simulink model "AEB_CodeGeneration"  (R2025a)
settings: Solver=VariableStepAuto  StartTime=0.0  StopTime=10.0  RelTol=1e-3
settings Model: Creator=Rudransh  LastModifiedBy=Rudransh

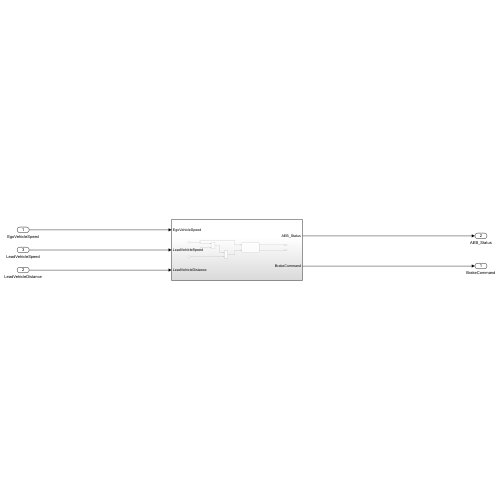
[thumbnail: Simulink's stored preview of the top-level diagram]
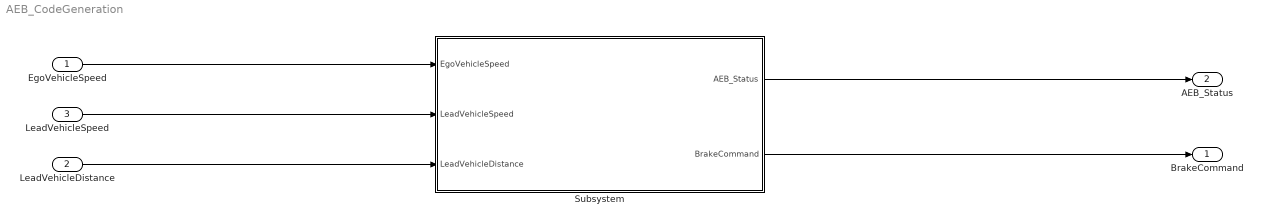
== system AEB_CodeGeneration ==
  EgoVehicleSpeed : Inport
  LeadVehicleDistance : Inport  Port=2
  LeadVehicleSpeed : Inport  Port=3
  Subsystem : Subsystem
  BrakeCommand : Outport
  AEB_Status : Outport  Port=2
  wires:
  EgoVehicleSpeed/1 -> Subsystem/1(EgoVehicleSpeed)
  LeadVehicleSpeed/1 -> Subsystem/2(LeadVehicleSpeed)
  LeadVehicleDistance/1 -> Subsystem/3(LeadVehicleDistance)
  Subsystem/1(AEB_Status) -> AEB_Status/1
  Subsystem/2(BrakeCommand) -> BrakeCommand/1

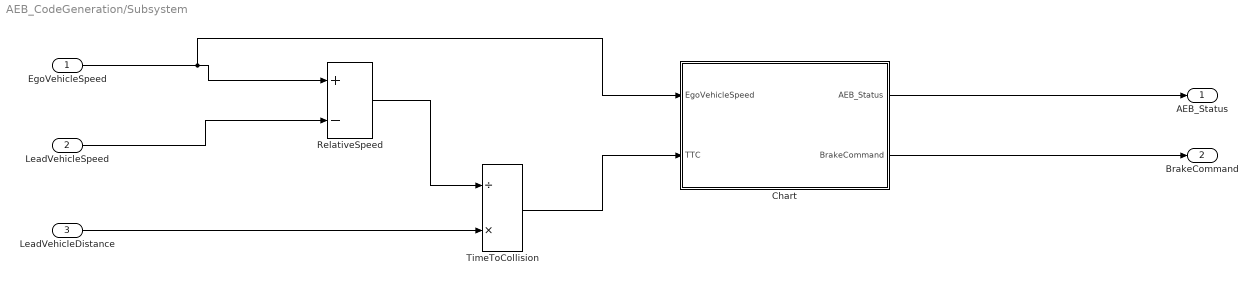
== system AEB_CodeGeneration/Subsystem ==
  EgoVehicleSpeed : Inport
  LeadVehicleSpeed : Inport  Port=2
  LeadVehicleDistance : Inport  Port=3
  Chart : Stateflow chart  TreatAsAtomicUnit=on
  RelativeSpeed : Sum  Inputs=+-
  TimeToCollision : Product  Inputs=/*
  AEB_Status : Outport
  BrakeCommand : Outport  Port=2
  wires:
  Chart/2(BrakeCommand) -> BrakeCommand/1
  Chart/1(AEB_Status) -> AEB_Status/1
  EgoVehicleSpeed/1 -> Chart/1(EgoVehicleSpeed), RelativeSpeed/1
  TimeToCollision/1 -> Chart/2(TTC)
  RelativeSpeed/1 -> TimeToCollision/1
  LeadVehicleSpeed/1 -> RelativeSpeed/2
  LeadVehicleDistance/1 -> TimeToCollision/2

== stateflow chart AEB_CodeGeneration/Subsystem/Chart ==
  state Safe
    entry: BrakeCommand = 0;
    AEB_Status = 0;
  state Warning
    entry: BrakeCommand = 0;
    AEB_Status = 1;
  state Braking
    entry: BrakeCommand = 1;
    AEB_Status = 2;
  (default) -> Safe
  Braking -> Safe : [EgoVehicleSpeed < 0.1]
  Safe -> Warning : [TTC < 2.5]
  Warning -> Safe [order 2] : [TTC >= 2.5]
  Warning -> Braking [order 1] : [TTC < 1.2]
  data: EgoVehicleSpeed input; AEB_Status output; BrakeCommand output; TTC input
